simulink model "Essai_CPU"  (R2019b)
settings: Solver=FixedStepAuto  StartTime=0.0  StopTime=inf  RelTol=1e-3  EnableMultiTasking=on
libraries: arduinolib x6, dspstat3 x2, simulink x1
settings Model: SILPILModeSetting=veronly  ExtModeTrigDuration=2  Creator=Etudiant  LastModifiedBy=Etudiant
settings OptimizationCC: EnhancedBackFolding=on  PassReuseOutputArgsAs=Individual arguments  ZeroExternalMemoryAtStartup=off  ZeroInternalMemoryAtStartup=off  MaxStackSize=64  OptimizeBlockOrder=speed  DifferentSizesBufferReuse=on  OptimizationCustomize=off  EfficientTunableParamExpr=on
settings DebuggingCC: ParameterPrecisionLossMsg=none  ParameterTunabilityLossMsg=error
settings HardwareCC: ProdBitPerInt=16  ProdBitPerPointer=16  ProdBitPerSizeT=16  ProdBitPerPtrDiffT=16  ProdLargestAtomicFloat=None  ProdWordSize=8  ProdHWDeviceType=Atmel->AVR
settings SFSimCC: MATLABDynamicMemAlloc=off
settings RTWCC: SystemTargetFile=ert.tlc  HardwareBoard=Arduino Mega 2560  TLCOptions=-aInlineSetEventsForThisBaseRateFcn=TLC_FALSE -aSuppressMultiTaskScheduler=TLC_FALSE -aRateBasedStepFcn=1  TemplateMakefile=ert_default_tmf  CustomSource=enc_eml_src.c  Toolchain=Arduino AVR  BuildConfiguration=Faster Runs  IncludeHyperlinkInReport=on
settings CodeAppCC: ForceParamTrailComments=on  GenerateComments=off  IgnoreCustomStorageClasses=off  OperatorAnnotations=on  SimulinkDataObjDesc=on  SFDataObjDesc=on  InsertBlockDesc=on
settings ERTTargetCC: SupportContinuousTime=on  SupportVariableSizeSignals=on  ExtModeStaticAllocSize=2048

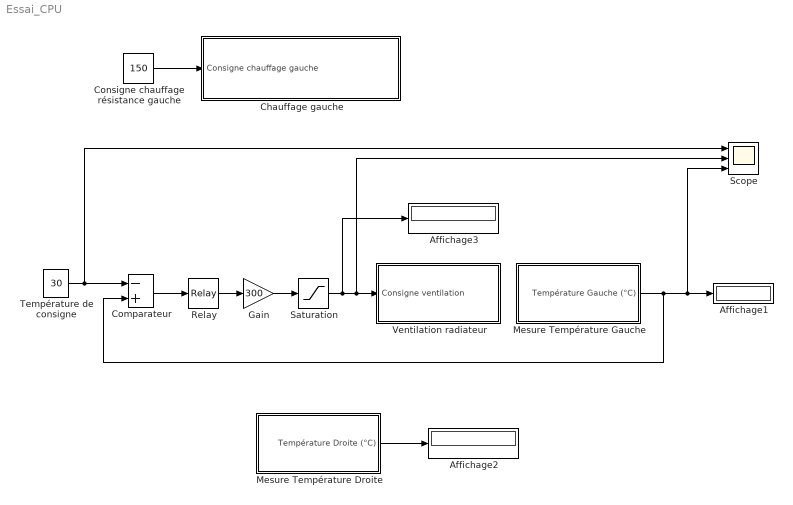
== system Essai_CPU ==
  Affichage1 : Display
  Affichage2 : Display
  Affichage3 : Display
  Chauffage gauche : Subsystem
  Comparateur : Sum  Inputs=-+  OutDataTypeStr=double
  Consigne chauffage résistance gauche : Constant  Value=150  SampleTime=-1
  Gain : Gain  Gain=300
  Mesure Température Droite : Subsystem
  Mesure Température Gauche : Subsystem
  Relay : Relay  OnSwitchValue=2  OffSwitchValue=0
  Saturation : Saturate  UpperLimit=255  LowerLimit=0
  Scope : Scope  NumInputPorts=3
  Température de consigne : Constant  Value=30  SampleTime=0.01
  Ventilation radiateur : Subsystem
  wires:
  Température de consigne/1 -> Scope/1, Comparateur/1
  Saturation/1 -> Affichage3/1, Scope/2, Ventilation radiateur/1(Consigne ventilation)
  Mesure Température Gauche/1(Température Gauche (°C)) -> Comparateur/2, Scope/3, Affichage1/1
  Comparateur/1 -> Relay/1
  Relay/1 -> Gain/1
  Gain/1 -> Saturation/1
  Consigne chauffage résistance gauche/1 -> Chauffage gauche/1(Consigne chauffage gauche)
  Mesure Température Droite/1(Température Droite (°C)) -> Affichage2/1

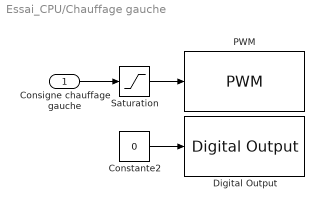
== system Essai_CPU/Chauffage gauche ==
  Consigne chauffage gauche : Inport
  Constante2 : Constant  Value=0  SampleTime=-1
  Digital Output : arduinolib/Digital Output  pinNumber=9  blockPlatform=arduino
  PWM : arduinolib/PWM  pinNumber=6  EnableInputFrequency=off  InitialFrequency=2000  InitialDutyCycle=0  NotificationType=None  blockPlatform=arduino
  Saturation : Saturate  UpperLimit=255  LowerLimit=0
  wires:
  Constante2/1 -> Digital Output/1
  Saturation/1 -> PWM/1
  Consigne chauffage gauche/1 -> Saturation/1

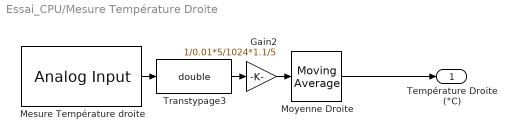
== system Essai_CPU/Mesure Température Droite ==
  Gain2 : Gain  Gain=1/0.01*5/1024*1.1/5
  Mesure Température droite : arduinolib/Analog Input  pinNumber=2  ReadResultsOnly=off  ConversionTriggerSource=Software  ExternalTriggerType=uint32(0)  OutputDataType=uint16  EnableConversionCompleteNotify=off  EnableOuputStatus=off  SampleTime=-1  blockPlatform=arduino
  Moyenne Droite : dspstat3/Moving Average  Method=Sliding window  ForgettingFactorPort=off  SpecifyWindowLength=on  WindowLength=5  ForgettingFactor=0.9  SimulateUsing=Code generation
  Transtypage3 : DataTypeConversion  OutDataTypeStr=double
  Température Droite (°C) : Outport
  wires:
  Gain2/1 -> Moyenne Droite/1
  Moyenne Droite/1 -> Température Droite (°C)/1
  Mesure Température droite/1 -> Transtypage3/1
  Transtypage3/1 -> Gain2/1

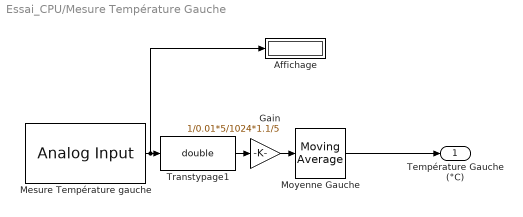
== system Essai_CPU/Mesure Température Gauche ==
  Affichage : Display
  Gain : Gain  Gain=1/0.01*5/1024*1.1/5
  Mesure Température gauche : arduinolib/Analog Input  pinNumber=0  ReadResultsOnly=off  ConversionTriggerSource=Software  ExternalTriggerType=uint32(0)  OutputDataType=uint16  EnableConversionCompleteNotify=off  EnableOuputStatus=off  SampleTime=-1  blockPlatform=arduino
  Moyenne Gauche : dspstat3/Moving Average  Method=Sliding window  ForgettingFactorPort=off  SpecifyWindowLength=on  WindowLength=5  ForgettingFactor=0.9  SimulateUsing=Code generation
  Transtypage1 : DataTypeConversion  OutDataTypeStr=double
  Température Gauche (°C) : Outport
  wires:
  Gain/1 -> Moyenne Gauche/1
  Mesure Température gauche/1 -> Affichage/1, Transtypage1/1
  Transtypage1/1 -> Gain/1
  Moyenne Gauche/1 -> Température Gauche (°C)/1

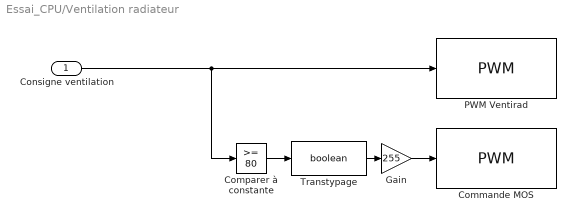
== system Essai_CPU/Ventilation radiateur ==
  Consigne ventilation : Inport
  Commande MOS : arduinolib/PWM  pinNumber=8  EnableInputFrequency=off  InitialFrequency=2000  InitialDutyCycle=0  NotificationType=None  blockPlatform=arduino
  Comparer à constante : simulink/Logic and Bit Operations/Compare To Constant  relop=>=  const=80  OutDataTypeStr=boolean
  Gain : Gain  Gain=255
  PWM Ventirad : arduinolib/PWM  pinNumber=12  EnableInputFrequency=off  InitialFrequency=2000  InitialDutyCycle=0  NotificationType=None  blockPlatform=arduino
  Transtypage : DataTypeConversion  OutDataTypeStr=boolean
  wires:
  Consigne ventilation/1 -> Comparer à constante/1, PWM Ventirad/1
  Transtypage/1 -> Gain/1
  Gain/1 -> Commande MOS/1
  Comparer à constante/1 -> Transtypage/1
